simulink model "model_po"  (Simulink 7.0)
settings: Solver=ode45  StartTime=0.0  StopTime=10.0  RelTol=1e-3
libraries: cstblocks x9
settings Model: Creator=fromion  LastModifiedBy=vfromion  ExtModeTrigMode=oneshot  ExtModeArmWhenConnect=off  ExtModeAutoUpdateStatusClock=off
settings DataIOCC: LimitDataPoints=off
settings OptimizationCC: BlockReduction=off  BooleanDataType=off
settings DebuggingCC: SaveWithParameterizedLinksMsg=none  SignalResolutionControl=TryResolveAllWithWarning  SolverPrmCheckMsg=none  MultiTaskDSMMsg=warning  MultiTaskCondExecSysMsg=none  StrictBusMsg=None
settings HardwareCC: TargetUnknown=on
settings RTWCC: IncludeERTFirstTime=on
settings GRTTargetCC: ModelReferenceCompliant=off  CompOptLevelCompliant=off  MatFileLogging=off

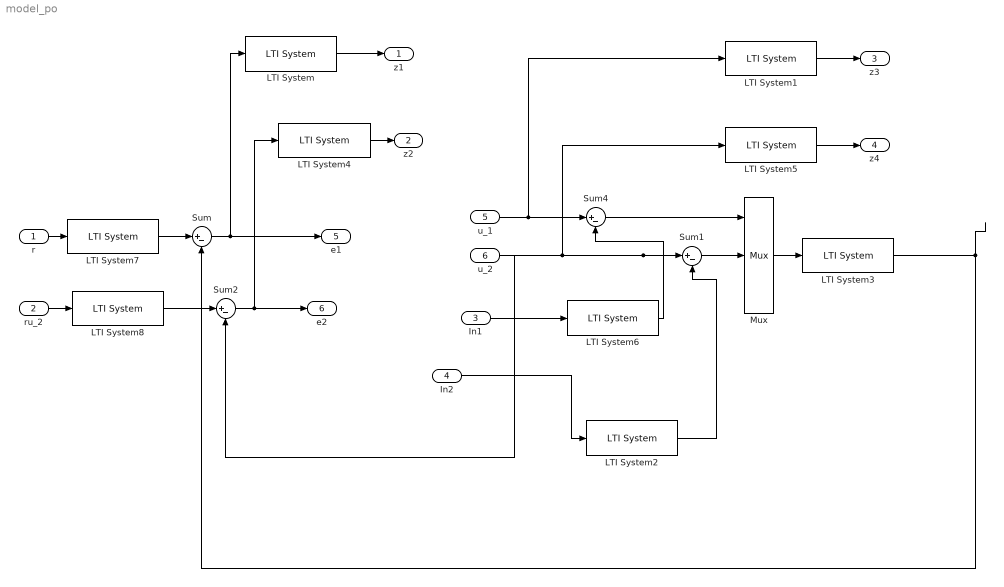
== system model_po ==
  r : Inport
  ru_2 : Inport  Port=2
  In1 : Inport  Port=3
  In2 : Inport  Port=4
  u_1 : Inport  Port=5
  u_2 : Inport  Port=6
  LTI System : cstblocks/LTI System  SystemSampleTime=-1  sys=W11  IC=0
  LTI System1 : cstblocks/LTI System  SystemSampleTime=-1  sys=W21  IC=0
  LTI System2 : cstblocks/LTI System  SystemSampleTime=-1  sys=Wp2  IC=0
  LTI System3 : cstblocks/LTI System  SystemSampleTime=-1  sys=sys_synt_ss  IC=0
  LTI System4 : cstblocks/LTI System  SystemSampleTime=-1  sys=W12  IC=0
  LTI System5 : cstblocks/LTI System  SystemSampleTime=-1  sys=W22  IC=0
  LTI System6 : cstblocks/LTI System  SystemSampleTime=-1  sys=Wp1  IC=0
  LTI System7 : cstblocks/LTI System  SystemSampleTime=-1  sys=Wpe1  IC=0
  LTI System8 : cstblocks/LTI System  SystemSampleTime=-1  sys=Wpe2  IC=0
  Mux : Mux  Inputs=3
  Sum{,1..2,4} (4 alike) : Sum  Inputs=|+-  SaturateOnIntegerOverflow=on  InputSameDT=on
  z1 : Outport
  z2 : Outport  Port=2
  z3 : Outport  Port=3
  z4 : Outport  Port=4
  e1 : Outport  Port=5
  e2 : Outport  Port=6
  wires:
  Sum/1 -> e1/1, LTI System/1
  LTI System1/1 -> z3/1
  In1/1 -> LTI System6/1
  r/1 -> LTI System7/1
  LTI System/1 -> z1/1
  LTI System3/1 -> Sum/2
  Sum4/1 -> Mux/1
  u_2/1 -> LTI System5/1, Sum1/1, Sum2/2
  LTI System5/1 -> z4/1
  LTI System6/1 -> Sum4/2
  In2/1 -> LTI System2/1
  LTI System2/1 -> Sum1/2
  ru_2/1 -> LTI System8/1
  Sum2/1 -> e2/1, LTI System4/1
  LTI System4/1 -> z2/1
  Mux/1 -> LTI System3/1
  u_1/1 -> Sum4/1, LTI System1/1
  Sum1/1 -> Mux/2
  LTI System7/1 -> Sum/1
  LTI System8/1 -> Sum2/1
